simulink model "TN2_Ziegler_Nichols_2"  (Simulink 7.4)
settings: Solver=ode45  StartTime=0.0  StopTime=10  RelTol=1e-3
settings Model: Creator=phuck  LastModifiedBy=Dell

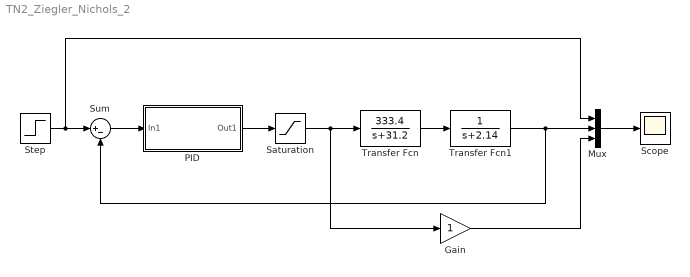
== system TN2_Ziegler_Nichols_2 ==
  Gain : Gain  ParameterDataType=fixdt(1, 16)  ParameterScaling=2^0  OutDataType=fixdt(1, 16)  OutScaling=2^0
  Mux : Mux  Inputs=3
  PID : Subsystem
  Saturation : Saturate  UpperLimit=30  LowerLimit=-30  OutDataType=fixdt(1, 16)  OutScaling=2^0
  Scope : Scope
      settings: TimeRange=0.001638400000000928  YMin=-30  YMax=110
  Step : Step  Time=0  After=100  SampleTime=0
  Sum : Sum  Inputs=|+-  OutDataType=fixdt(1, 16)  OutScaling=2^0
  Transfer Fcn : TransferFcn  Numerator=[333.4]  Denominator=[1 31.2]
  Transfer Fcn1 : TransferFcn  Denominator=[1 2.14]
  wires:
  Saturation/1 -> Gain/1, Transfer Fcn/1
  Step/1 -> Sum/1, Mux/1
  Sum/1 -> PID/1(In1)
  Mux/1 -> Scope/1
  Gain/1 -> Mux/3
  Transfer Fcn/1 -> Transfer Fcn1/1
  Transfer Fcn1/1 -> Mux/2, Sum/2
  PID/1(Out1) -> Saturation/1

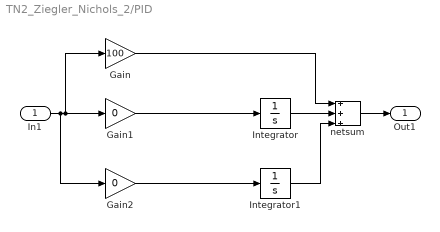
== system TN2_Ziegler_Nichols_2/PID ==
  In1 : Inport  OutDataType=fixdt(1, 16)  OutScaling=2^0
  Gain : Gain  Gain=100  ParameterDataType=fixdt(1, 16)  ParameterScaling=2^0  OutDataType=fixdt(1, 16)  OutScaling=2^0
  Gain1 : Gain  Gain=0  ParameterDataType=fixdt(1, 16)  ParameterScaling=2^0  OutDataType=fixdt(1, 16)  OutScaling=2^0
  Gain2 : Gain  Gain=0  ParameterDataType=fixdt(1, 16)  ParameterScaling=2^0  OutDataType=fixdt(1, 16)  OutScaling=2^0
  Integrator : Integrator
  Integrator1 : Integrator
  netsum : Sum  Inputs=3  OutDataType=sfix(16)  OutScaling=2^0  SaturateOnIntegerOverflow=on  InputSameDT=on  OutDataTypeStr=Inherit: Same as first input
  Out1 : Outport  OutDataType=fixdt(1, 16)  OutScaling=2^0
  wires:
  In1/1 -> Gain1/1, Gain/1, Gain2/1
  Gain/1 -> netsum/1
  Gain1/1 -> Integrator/1
  Integrator/1 -> netsum/2
  netsum/1 -> Out1/1
  Integrator1/1 -> netsum/3
  Gain2/1 -> Integrator1/1
